simulink model "F16version1"  (R2023b)
settings: Solver=VariableStepAuto  StartTime=0.0  StopTime=60  FixedStep=0.1  RelTol=1e-3
libraries: simulink_extras x4, simulink x2, aerolibasang x2, shared6dof x1, aerolibanim x1
(part 2 of 2)

== matlab function F16version1/Subsystem/Subsystem1/MATLAB Function2 ==
  data: alpha input; c_m output; el input
function c_m = compute_cm_fixed(alpha, el)
    % Embedded data
    data_CM_updated_data_full = [
        0.205, 0.168, 0.186, 0.196, 0.213, 0.251, 0.245, 0.238, 0.252, 0.231, 0.198, 0.192;
        0.081, 0.077, 0.107, 0.110, 0.110, 0.141, 0.127, 0.119, 0.133, 0.108, 0.081, 0.093;
        -0.046, -0.020, -0.009, -0.005, -0.006, 0.010, 0.006, -0.001, 0.014, 0.000, -0.013, 0.032;
        -0.174, -0.145, -0.121, -0.127, -0.129, -0.102, -0.097, -0.113, -0.087, -0.084, -0.069, -0.006;
        -0.259, -0.202, -0.184, -0.193, -0.199, -0.150, -0.160, -0.167, -0.104, -0.076, -0.041, -0.005
    ];

    % Map Alpha and EL into indices and interpolate
    scaled_alpha = 0.2 * alpha;
    k = floor(scaled_alpha);
    k = max(-2, min(k, 8)); % Constrain within bounds
    da = scaled_alpha - k;
    l = k + sign(1.1 * da);
    l = max(-1, min(l, 8)); % Constrain within bounds

    % Adjust indices for MATLAB (1-based indexing)
    k_index = k + 3;
    l_index = l + 3;

    scaled_el = el / 12.5;
    m = floor(scaled_el);
    m = max(-2, min(m, 2)); % Constrain within bounds
    de = scaled_el - m;
    n = m + sign(1.1 * de);
    n = max(-2, min(n, 2)); % Constrain within bounds

    % Adjust indices for MATLAB (1-based indexing)
    m_index = m + 3;
    n_index = n + 3;

    % Interpolate values
    t = data_CM_updated_data_full(m_index, k_index);
    u = data_CM_updated_data_full(n_index, k_index);
    v = t + abs(da) * (data_CM_updated_data_full(m_index, l_index) - t);
    w = u + abs(da) * (data_CM_updated_data_full(n_index, l_index) - u);

    % Final interpolation
    c_m = v + (w - v) * abs(de);
end

== matlab function F16version1/Subsystem/Subsystem1/MATLAB Function3 ==
  data: alpha input; c_l output; beta input
function c_l = compute_cl_fixed(alpha, beta)
    % Embedded data
    data_CL_updated_data_full = [
        -0.001, -0.004, -0.008, -0.012, -0.016, -0.019, -0.020, -0.020, -0.015, -0.008, -0.013, -0.015;
        -0.003, -0.009, -0.017, -0.024, -0.030, -0.034, -0.040, -0.037, -0.016, -0.002, -0.010, -0.019;
        -0.001, -0.010, -0.020, -0.030, -0.039, -0.044, -0.050, -0.049, -0.023, -0.006, -0.014, -0.027;
        0.000, -0.010, -0.022, -0.034, -0.047, -0.046, -0.059, -0.061, -0.033, -0.036, -0.035, -0.035;
        0.007, -0.010, -0.023, -0.034, -0.049, -0.046, -0.068, -0.071, -0.060, -0.058, -0.062, -0.059;
        0.009, -0.011, -0.023, -0.037, -0.050, -0.047, -0.074, -0.079, -0.091, -0.076, -0.077, -0.076
    ];

    % Scale and map alpha into indices
    scaled_alpha = 0.2 * alpha;
    k = floor(scaled_alpha);                  % Find lower index
    k = max(-2, min(k, 8));                   % Constrain within bounds
    da = scaled_alpha - k;                    % Fractional part for interpolation
    l = k + sign(1.1 * da);                   % Find upper index
    l = max(-2, min(l, 8));                   % Constrain within bounds

    % Adjust indices for MATLAB (1-based indexing)
    k_index = k + 3;                          % Shift index for 1-based indexing
    l_index = l + 3;                          % Shift index for 1-based indexing

    % Scale and map beta into indices
    scaled_beta = 0.2 * abs(beta);
    m = floor(scaled_beta);                   % Find lower index
    m = max(0, min(m, 5));                    % Constrain within bounds
    db = scaled_beta - m;                     % Fractional part for interpolation
    n = m + sign(1.1 * db);                   % Find upper index
    n = max(0, min(n, 5));                    % Constrain within bounds

    % Adjust indices for MATLAB (1-based indexing)
    m_index = m + 1;                          % Shift index for 1-based indexing
    n_index = n + 1;                          % Shift index for 1-based indexing

    % Interpolation in the alpha dimension
    t = data_CL_updated_data_full(m_index, k_index); % Lower beta, lower alpha
    u = data_CL_updated_data_full(n_index, k_index); % Upper beta, lower alpha
    v = t + abs(da) * (data_CL_updated_data_full(m_index, l_index) - t); % Lower beta, interpolated alpha
    w = u + abs(da) * (data_CL_updated_data_full(n_index, l_index) - u); % Upper beta, interpolated alpha

    % Interpolation in the beta dimension
    c_l = v + (w - v) * abs(db);              % Final interpolated value
end

== matlab function F16version1/Subsystem/Subsystem1/MATLAB Function4 ==
  data: alpha input; c_n output; beta input
function c_n = compute_cn_fixed(alpha, beta)
    % Embedded data
    data_CN_updated_data_full = [
        0.018, 0.019, 0.018, 0.019, 0.019, 0.018, 0.013, 0.007, 0.004, -0.014, -0.017, -0.033;
        0.038, 0.042, 0.042, 0.042, 0.043, 0.039, 0.030, 0.017, 0.004, -0.035, -0.047, -0.057;
        0.056, 0.057, 0.059, 0.058, 0.058, 0.053, 0.032, 0.012, 0.002, -0.046, -0.071, -0.073;
        0.064, 0.077, 0.076, 0.074, 0.073, 0.057, 0.029, 0.007, 0.012, -0.034, -0.065, -0.041;
        0.074, 0.086, 0.093, 0.089, 0.080, 0.062, 0.049, 0.022, 0.028, -0.012, -0.002, -0.013;
        0.079, 0.090, 0.106, 0.106, 0.096, 0.080, 0.068, 0.030, 0.064, 0.015, 0.011, -0.001
    ];

    % Scale and map alpha into indices
    scaled_alpha = 0.2 * alpha;
    k = floor(scaled_alpha);                  % Find lower index
    k = max(-2, min(k, 8));                   % Constrain within bounds
    da = scaled_alpha - k;                    % Fractional part for interpolation
    l = k + sign(1.1 * da);                   % Find upper index
    l = max(-2, min(l, 8));                   % Constrain within bounds

    % Adjust indices for MATLAB (1-based indexing)
    k_index = k + 3;                          % Shift index for 1-based indexing
    l_index = l + 3;                          % Shift index for 1-based indexing

    % Scale and map beta into indices
    scaled_beta = 0.2 * abs(beta);
    m = floor(scaled_beta);                   % Find lower index
    m = max(0, min(m, 5));                    % Constrain within bounds
    db = scaled_beta - m;                     % Fractional part for interpolation
    n = m + sign(1.1 * db);                   % Find upper index
    n = max(0, min(n, 5));                    % Constrain within bounds

    % Adjust indices for MATLAB (1-based indexing)
    m_index = m + 1;                          % Shift index for 1-based indexing
    n_index = n + 1;                          % Shift index for 1-based indexing

    % Interpolation in the alpha dimension
    t = data_CN_updated_data_full(m_index, k_index); % Lower beta, lower alpha
    u = data_CN_updated_data_full(n_index, k_index); % Upper beta, lower alpha
    v = t + abs(da) * (data_CN_updated_data_full(m_index, l_index) - t); % Lower beta, interpolated alpha
    w = u + abs(da) * (data_CN_updated_data_full(n_index, l_index) - u); % Upper beta, interpolated alpha

    % Interpolation in the beta dimension
    c_n = v + (w - v) * abs(db);              % Final interpolated value
end

== matlab function F16version1/Subsystem/Subsystem1/MATLAB Function5 ==
  data: Beta input; c_y output; AIL input; RDR input
function c_y = compute_C_Y(Beta, AIL, RDR)
    % Compute C_Y based on Beta, AIL, and RDR
    c_y = (-0.02) * Beta + (0.021) * (AIL / 20.0) + (0.086) * (RDR / 30.0);
end

== matlab function F16version1/Subsystem/Subsystem/MATLAB Function ==
  data: U input; V_t output; V input; W input; alpha output; beta output
function [V_t, alpha, beta] = fcn(U, V, W)
    % Calculate the total velocity V_t
    V_t = sqrt(U^2 + V^2 + W^2);
    
    % Calculate alpha (angle of attack)
    % alpha = atan(W / U);
    alpha = atan2(W,U);
    % alpha = 0.698;
    
    % Calculate beta (side slip angle)
    % beta = atan(V / V_t);
    beta = asin(V / V_t);

    
    % Return the values
    % No need for 'y = V_t, alpha, beta;' as we already specify output variables
end

== matlab function F16version1/Subsystem2/MATLAB Function ==
  data: U input; V_t output; V input; W input; alpha output; beta output
function [V_t, alpha, beta] = fcn(U, V, W)
    % Calculate the total velocity V_t
    V_t = sqrt(U^2 + V^2 + W^2);
    
    % Calculate alpha (angle of attack)
    alpha = atan2(W , U);
    % alpha = 0.698;
    
    % Calculate beta (side slip angle)
    beta = asin(V / V_t);
    % beta = atan(V / V_t);
    
    % Return the values
    % No need for 'y = V_t, alpha, beta;' as we already specify output variables
end

== matlab function F16version1/MATLAB Function ==
  data: alpha input; c_x output; el input
function c_x = compute_cx_fixed(alpha, el)
    data = [
    -0.099, -0.081, -0.081, -0.063, -0.025, 0.044, 0.097, 0.113, 0.145, 0.167, 0.174, 0.166;
    -0.048, -0.038, -0.040, -0.021, 0.016, 0.083, 0.127, 0.137, 0.162, 0.177, 0.179, 0.167;
    -0.022, -0.020, -0.021, -0.004, 0.032, 0.094, 0.128, 0.130, 0.154, 0.161, 0.155, 0.138;
    -0.040, -0.038, -0.039, -0.025, 0.006, 0.062, 0.087, 0.085, 0.100, 0.110, 0.104, 0.091;
    -0.083, -0.073, -0.076, -0.072, -0.046, 0.012, 0.024, 0.025, 0.043, 0.053, 0.047, 0.040
    ];
    % Scale Alpha and EL
    scaled_alpha = 0.2 * alpha;
    k = floor(scaled_alpha);
    k = max(-2, min(k, 8)); % Constrain within bounds
    da = scaled_alpha - k;
    l = k + sign(1.1 * da);
    l = max(-2, min(l, 8)); % Constrain within bounds

    % Adjust indices for 1-based indexing
    k_index = k + 3; % MATLAB 1-based (add 3 instead of 2 for [-2, 8])
    l_index = l + 3;

    % Scale EL
    scaled_el = el / 12.5;
    m = floor(scaled_el);
    m = max(-2, min(m, 2)); % Constrain within bounds
    de = scaled_el - m;
    n = m + sign(1.1 * de);
    n = max(-2, min(n, 2)); % Constrain within bounds

    % Adjust indices for 1-based indexing
    m_index = m + 3; % MATLAB 1-based (add 3 instead of 2 for [-2, 2])
    n_index = n + 3;

    % Ensure indices are within valid ranges
    assert(m_index >= 1 && m_index <= size(data, 1), 'm_index out of bounds');
    assert(n_index >= 1 && n_index <= size(data, 1), 'n_index out of bounds');
    assert(k_index >= 1 && k_index <= size(data, 2), 'k_index out of bounds');
    assert(l_index >= 1 && l_index <= size(data, 2), 'l_index out of bounds');

    % Interpolate values
    t = data(m_index, k_index); % Top-left
    u = data(n_index, k_index); % Bottom-left
    v = t + abs(da) * (data(m_index, l_index) - t); % Interpolation along top row
    w = u + abs(da) * (data(n_index, l_index) - u); % Interpolation along bottom row
    c_x = v + (w - v) * abs(de); % Final interpolation
end

== matlab function F16version1/MATLAB Function1 ==
  data: alpha input; c_z output; beta input; el input


function c_z = compute_cz(alpha, beta, el)
    data_CZ_updated_data_full = [
    0.770, 0.241, -0.100, -0.416, -0.731, -1.053, ...
    -1.366, -1.646, -1.917, -2.120, -2.248, -2.229
    ];
    
    % Map Alpha into indices and interpolate
    scaled_alpha = 0.2 * alpha;
    k = floor(scaled_alpha);
    k = max(-2, min(k, 8)); % Constrain within bounds
    da = scaled_alpha - k;
    l = k + sign(1.1 * da);
    l = max(-1, min(l, 8)); % Constrain within bounds

    % Adjust index for MATLAB (1-based indexing)
    k_index = k + 3;
    l_index = l + 3;

    % Calculate 's' using the provided formula
    s = data_CZ_updated_data_full(k_index) + abs(da) * ...
        (data_CZ_updated_data_full(l_index) - data_CZ_updated_data_full(k_index));
    c_z = s * (1 - (beta / 57.3)^2) - 0.19 * (el / 25.0);
end
